simulink library "qrd_matrix_library"  (Simulink 8.7)
settings: Solver=ode45  StartTime=0.0  StopTime=10.0  RelTol=1e-3
values from neighbouring files (symbols this model uses):
  vectorization = 2    [qrd_test.m]
undefined symbols (not defined in the file or in its folder): AdvDSPBChannelOutDisplay, AdvDSPBDMemDisplay, Back_Substitution_instances, column_count, column_count_1, column_count_2, dpoly, dspba_ChannelInVis, dspba_ChannelOutVis, dspba_internal_get_channel_ports, evalAionMaskParam, latency, primtype, QRD_vectorization, recipsqrt, row, row_count, row_count_1, row_count_2, UseDontCare, value, x
libraries: DSPBAPrim x683, DSPBAControl x37, qrd_matrix_library x33, DSPBAVectorUtil x6, DSPBAVectorPrim x3
(part 8 of 8)

== system qrd_matrix_library/matrix_inversion/Z_Address_Gen ==
  Valid_In : Inport
  Channel_In : Inport  Port=2
  Minor_Index : Inport  Port=3
  Major_Index : Inport  Port=4
  size : Inport  Port=5
  SOP_In : Inport  Port=6
  EOP_In : Inport  Port=7
  Add : DSPBAPrim/Add  primtype=add  nInputs=evalAionMaskParam(gcb,'value',1)  nOutputs=1  omode=Specify via dialog  otype=uint(nextpow2(size*size/vectorization))  scale=1  rndmethod=Unbiased  factor=1  satmethod=Symmetric  shift_vec=[0 1 2 -1]  value=2  inPortNames=[' '; ' ';]  outPortNames=[' ']  dspbaimage=dspba_prim.jpg  text=fprintf('+');  style=Optimised  visibilities=1032+2^17+2^18+2^19  genFPC=off  floatRounding=correct  advOptions=[]  version=20130821
  ChannelIn : DSPBAPrim/ChannelIn  primtype=channelin  nInputs=dspba_internal_get_channel_ports(gcb)  nOutputs=dspba_internal_get_channel_ports(gcb)  omode=Inherit via internal rule  otype=sfix(16)  scale=2^-15  rndmethod=Unbiased  factor=1  satmethod=Symmetric  shift_vec=[0 1 2 -1]  value=5  inPortNames=['v'; 'c'; '0'; '1'; '2'; '3'; '4'; '5'; '6'; '7'; '8'; '9'; 'A'; 'B'; 'D'; 'E'; 'F'; 'G'; 'H'; 'I'; 'J'; 'K'; 'L'; 'M'; 'N'; 'O'; 'P'; 'Q'; 'R'; 'S'; 'T'; 'U'; 'W'; 'X'; 'Y'; 'Z']  outPortNames=['v'; 'c'; '0'; '1'; '2'; '3'; '4'; '5'; '6'; '7'; '8'; '9'; 'A'; 'B'; 'D'; 'E'; 'F'; 'G'; 'H'; 'I'; 'J'; 'K'; 'L'; 'M'; 'N'; 'O'; 'P'; 'Q'; 'R'; 'S'; 'T'; 'U'; 'W'; 'X'; 'Y'; 'Z']  dspbaimage=dspba_prim.jpg  text=fprintf('In');  style=Optimised  dataSignals=5  foldingEnabled=off  channels=1  sampleRate=200  packetBeginPresent=off  packetBeginEnabled=off  visibilities=dspba_ChannelInVis(gcb)  latencyCorrection=0  version=20141013
  ChannelOut : DSPBAPrim/ChannelOut  primtype=channelout  nInputs=dspba_internal_get_channel_ports(gcb)  nOutputs=dspba_internal_get_channel_ports(gcb)  omode=Inherit via internal rule  otype=sfix(16)  scale=2^-15  rndmethod=Unbiased  factor=1  satmethod=Symmetric  shift_vec=[0 1 2 -1]  value=3  inPortNames=['v'; 'c'; '0'; '1'; '2'; '3'; '4'; '5'; '6'; '7'; '8'; '9'; 'A'; 'B'; 'D'; 'E'; 'F'; 'G'; 'H'; 'I'; 'J'; 'K'; 'L'; 'M'; 'N'; 'O'; 'P'; 'Q'; 'R'; 'S'; 'T'; 'U'; 'W'; 'X'; 'Y'; 'Z']  outPortNames=['v'; 'c'; '0'; '1'; '2'; '3'; '4'; '5'; '6'; '7'; '8'; '9'; 'A'; 'B'; 'D'; 'E'; 'F'; 'G'; 'H'; 'I'; 'J'; 'K'; 'L'; 'M'; 'N'; 'O'; 'P'; 'Q'; 'R'; 'S'; 'T'; 'U'; 'W'; 'X'; 'Y'; 'Z']  dspbaimage=dspba_prim.jpg  text=fprintf('Out%s', AdvDSPBChannelOutDisplay(latency));  style=Optimised  dataSignals=3  foldingEnabled=off  channels=1  sampleRate=200  packetBeginPresent=off  packetBeginEnabled=off  visibilities=dspba_ChannelOutVis(gcb)  latency=0  latencyCorrection=0  version=20141013
  Mult : DSPBAPrim/Mult  primtype=mult  nInputs=2  nOutputs=1  omode=Inherit via internal rule  otype=sfix(16)  scale=2^-15  rndmethod=Unbiased  factor=1  satmethod=Symmetric  shift_vec=[0 1 2 -1]  value=0  inPortNames=[' '; ' ';]  outPortNames=[' ']  dspbaimage=dspba_prim.jpg  text=fprintf('X');  style=Optimised  visibilities=8+2^18+2^19  floatPrecision=float32_m23  floatRounding=correct  advOptions=[]  version=20130115
  SynthesisInfo : DSPBAPrim/SynthesisInfo  primtype=synthinfo  nInputs=0  nOutputs=0  omode=Inherit via internal rule  otype=sfix(16)  scale=2^-15  rndmethod=Truncate  factor=1  satmethod=Symmetric  shift_vec=[0 1 2 -1]  value=99  inPortNames=[' '; ' ';]  outPortNames=[' ']  dspbaimage=dspba_prim_ctrl.jpg  text=fprintf('Style=%s', style);  style=Scheduled  visibilities=32768  constraintInUse=off  constraintRelation=>  constraintLimit=2  bitAccurate=off  version=20150220
  Valid_Out : Outport
  Channel_Out : Outport  Port=2
  Read_Address : Outport  Port=3
  SOP_Out : Outport  Port=4
  EOP_Out : Outport  Port=5
  wires:
  ChannelIn/2 -> ChannelOut/2
  ChannelOut/5 -> EOP_Out/1
  ChannelOut/4 -> SOP_Out/1
  EOP_In/1 -> ChannelIn/7
  SOP_In/1 -> ChannelIn/6
  ChannelIn/7 -> ChannelOut/5
  ChannelIn/6 -> ChannelOut/4
  Add/1 -> ChannelOut/3
  ChannelIn/5 -> Mult/2
  size/1 -> ChannelIn/5
  Major_Index/1 -> ChannelIn/4
  ChannelOut/2 -> Channel_Out/1
  ChannelOut/3 -> Read_Address/1
  ChannelOut/1 -> Valid_Out/1
  ChannelIn/3 -> Mult/1
  Mult/1 -> Add/2
  ChannelIn/1 -> ChannelOut/1
  Channel_In/1 -> ChannelIn/2
  Minor_Index/1 -> ChannelIn/3
  Valid_In/1 -> ChannelIn/1
  ChannelIn/4 -> Add/1

== system qrd_matrix_library/matrix_inversion/vectorizer ==
  Valid_In : Inport
  Channel_In : Inport  Port=2
  Data_In : Inport  Port=3
  SOP_In : Inport  Port=4
  EOP_In : Inport  Port=5
  ChannelIn : DSPBAPrim/ChannelIn  Commented=on  primtype=channelin  nInputs=dspba_internal_get_channel_ports(gcb)  nOutputs=dspba_internal_get_channel_ports(gcb)  omode=Inherit via internal rule  otype=sfix(16)  scale=2^-15  rndmethod=Unbiased  factor=1  satmethod=Symmetric  shift_vec=[0 1 2 -1]  value=3  inPortNames=['v'; 'c'; '0'; '1'; '2'; '3'; '4'; '5'; '6'; '7'; '8'; '9'; 'A'; 'B'; 'D'; 'E'; 'F'; 'G'; 'H'; 'I'; 'J'; 'K'; 'L'; 'M'; 'N'; 'O'; 'P'; 'Q'; 'R'; 'S'; 'T'; 'U'; 'W'; 'X'; 'Y'; 'Z']  outPortNames=['v'; 'c'; '0'; '1'; '2'; '3'; '4'; '5'; '6'; '7'; '8'; '9'; 'A'; 'B'; 'D'; 'E'; 'F'; 'G'; 'H'; 'I'; 'J'; 'K'; 'L'; 'M'; 'N'; 'O'; 'P'; 'Q'; 'R'; 'S'; 'T'; 'U'; 'W'; 'X'; 'Y'; 'Z']  dspbaimage=dspba_prim.jpg  text=fprintf('In');  style=Optimised  dataSignals=3  foldingEnabled=off  channels=1  sampleRate=200  packetBeginPresent=off  packetBeginEnabled=off  visibilities=dspba_ChannelInVis(gcb)  latencyCorrection=0  version=20141013
  ChannelOut : DSPBAPrim/ChannelOut  Commented=on  primtype=channelout  nInputs=dspba_internal_get_channel_ports(gcb)  nOutputs=dspba_internal_get_channel_ports(gcb)  omode=Inherit via internal rule  otype=sfix(16)  scale=2^-15  rndmethod=Unbiased  factor=1  satmethod=Symmetric  shift_vec=[0 1 2 -1]  value=3  inPortNames=['v'; 'c'; '0'; '1'; '2'; '3'; '4'; '5'; '6'; '7'; '8'; '9'; 'A'; 'B'; 'D'; 'E'; 'F'; 'G'; 'H'; 'I'; 'J'; 'K'; 'L'; 'M'; 'N'; 'O'; 'P'; 'Q'; 'R'; 'S'; 'T'; 'U'; 'W'; 'X'; 'Y'; 'Z']  outPortNames=['v'; 'c'; '0'; '1'; '2'; '3'; '4'; '5'; '6'; '7'; '8'; '9'; 'A'; 'B'; 'D'; 'E'; 'F'; 'G'; 'H'; 'I'; 'J'; 'K'; 'L'; 'M'; 'N'; 'O'; 'P'; 'Q'; 'R'; 'S'; 'T'; 'U'; 'W'; 'X'; 'Y'; 'Z']  dspbaimage=dspba_prim.jpg  text=fprintf('Out%s', AdvDSPBChannelOutDisplay(latency));  style=Optimised  dataSignals=3  foldingEnabled=off  channels=1  sampleRate=200  packetBeginPresent=off  packetBeginEnabled=off  visibilities=dspba_ChannelOutVis(gcb)  latency=0  latencyCorrection=0  version=20141013
  CmpEQ : DSPBAPrim/CmpEQ  primtype=cmpeq  nInputs=2  nOutputs=1  omode=boolean  otype=sfix(16)  scale=2^-15  rndmethod=Unbiased  factor=1  satmethod=Symmetric  shift_vec=[0 1 2 -1]  value=0  inPortNames=[' '; ' ';]  outPortNames=[' ']  dspbaimage=dspba_prim.jpg  text=fprintf('==');  style=Optimised  visibilities=0  advOptions=[]  version=20130117
  Const1 : DSPBAPrim/Const  primtype=const  nInputs=0  nOutputs=1  omode=Inherit via internal rule  otype=uint(8)  scale=1  rndmethod=Unbiased  factor=1  satmethod=Symmetric  shift_vec=[0 1 2 -1]  value=1  inPortNames=['+'; '+';]  outPortNames=[' ']  dspbaimage=dspba_prim.jpg  text=fprintf('%s', num2str(value));  style=Optimised  visibilities=8 + 1024  floatPrecision=float32_m23  version=20120820
  Const11 : DSPBAPrim/Const  primtype=const  nInputs=0  nOutputs=1  omode=Inherit via internal rule  otype=uint(8)  scale=1  rndmethod=Unbiased  factor=1  satmethod=Symmetric  shift_vec=[0 1 2 -1]  value=Back_Substitution_instances/QRD_vectorization  inPortNames=['+'; '+';]  outPortNames=[' ']  dspbaimage=dspba_prim.jpg  text=fprintf('%s', num2str(value));  style=Optimised  visibilities=8 + 1024  floatPrecision=float32_m23  version=20120820
  Const2 : DSPBAPrim/Const  primtype=const  nInputs=0  nOutputs=1  omode=Inherit via internal rule  otype=uint(8)  scale=1  rndmethod=Unbiased  factor=1  satmethod=Symmetric  shift_vec=[0 1 2 -1]  value=(Back_Substitution_instances/QRD_vectorization)-1  inPortNames=['+'; '+';]  outPortNames=[' ']  dspbaimage=dspba_prim.jpg  text=fprintf('%s', num2str(value));  style=Optimised  visibilities=8 + 1024  floatPrecision=float32_m23  version=20120820
  Const8 : DSPBAPrim/Const  primtype=const  nInputs=0  nOutputs=1  omode=Inherit via internal rule  otype=uint(8)  scale=1  rndmethod=Unbiased  factor=1  satmethod=Symmetric  shift_vec=[0 1 2 -1]  value=0  inPortNames=['+'; '+';]  outPortNames=[' ']  dspbaimage=dspba_prim.jpg  text=fprintf('%s', num2str(value));  style=Optimised  visibilities=8 + 1024  floatPrecision=float32_m23  version=20120820
  LoadableCounter : DSPBAPrim/LoadableCounter  primtype=loadablecounter  nInputs=5  nOutputs=1  omode=Inherit via internal rule  otype=ufix(16)  scale=2^-0  rndmethod=Unbiased  factor=1  satmethod=Symmetric  shift_vec=[0 1 2 -1]  value=[0 (Back_Substitution_instances/QRD_vectorization) 0]  inPortNames=['en';'ld';'i ';'s ';'m ']  outPortNames=[' ']  dspbaimage=dspba_prim.jpg  text=fprintf('loadable\ncounter\n[%d %d %d]', value(1), value(2), value(3));  style=Optimised  visibilities=8 + 1024  version=20090407
  SynthesisInfo : DSPBAPrim/SynthesisInfo  Commented=on  primtype=synthinfo  nInputs=0  nOutputs=0  omode=Inherit via internal rule  otype=sfix(16)  scale=2^-15  rndmethod=Truncate  factor=1  satmethod=Symmetric  shift_vec=[0 1 2 -1]  value=99  inPortNames=[' '; ' ';]  outPortNames=[' ']  dspbaimage=dspba_prim_ctrl.jpg  text=fprintf('Style=%s', style);  style=Scheduled  visibilities=2^17+2^18+2^19+2^20  constraintInUse=off  constraintRelation=>  constraintLimit=2  bitAccurate=off  version=20150220
  TappedDelay : qrd_matrix_library/TappedDelay  numTaps=Back_Substitution_instances/QRD_vectorization
  cmp_delay{,1..4} (5 alike) : DSPBAPrim/SampleDelay  primtype=sampdelay  nInputs=1  nOutputs=1  omode=Inherit via internal rule  otype=sfix(16)  scale=2^-15  rndmethod=Unbiased  factor=1  satmethod=Symmetric  shift_vec=[0 1 2 -1]  value=1  inPortNames=[' '; ' ';]  outPortNames=[' ']  dspbaimage=dspba_prim.jpg  text=dpoly(1, eye(1,value+1), 'z')  style=Optimised  visibilities=8 + 1024 + 2^17 + 2^18  flexible=off  slackgroup=0  augmented=0  version=20090407  advOptions=[]
  cntdelay{,1..4} (5 alike) : DSPBAPrim/SampleDelay  primtype=sampdelay  nInputs=1  nOutputs=1  omode=Inherit via internal rule  otype=sfix(16)  scale=2^-15  rndmethod=Unbiased  factor=1  satmethod=Symmetric  shift_vec=[0 1 2 -1]  value=(Back_Substitution_instances/QRD_vectorization)-1  inPortNames=[' '; ' ';]  outPortNames=[' ']  dspbaimage=dspba_prim.jpg  text=dpoly(1, eye(1,value+1), 'z')  style=Optimised  visibilities=8 + 1024 + 2^17 + 2^18  flexible=off  slackgroup=0  augmented=0  version=20090407  advOptions=[]
  sop_delay : DSPBAPrim/SampleDelay  primtype=sampdelay  nInputs=1  nOutputs=1  omode=Inherit via internal rule  otype=sfix(16)  scale=2^-15  rndmethod=Unbiased  factor=1  satmethod=Symmetric  shift_vec=[0 1 2 -1]  value=(Back_Substitution_instances/QRD_vectorization)-1  inPortNames=[' '; ' ';]  outPortNames=[' ']  dspbaimage=dspba_prim.jpg  text=dpoly(1, eye(1,value+1), 'z')  style=Optimised  visibilities=8 + 1024 + 2^17 + 2^18  flexible=off  slackgroup=0  augmented=0  version=20090407  advOptions=[]
  Valid_Out : Outport
  Channel_Out : Outport  Port=2
  Data_Out : Outport  Port=3
  SOP_Out : Outport  Port=4
  EOP_Out : Outport  Port=5
  wires:
  CmpEQ/1 -> cmp_delay/1
  TappedDelay/1 -> cmp_delay2/1
  cntdelay4/1 -> cmp_delay4/1
  cntdelay1/1 -> cmp_delay1/1
  cntdelay3/1 -> sop_delay/1
  LoadableCounter/1 -> CmpEQ/1
  Valid_In/1 -> cntdelay/1
  Channel_In/1 -> cntdelay1/1
  Data_In/1 -> cntdelay2/1
  SOP_In/1 -> cntdelay3/1, LoadableCounter/2
  EOP_In/1 -> cntdelay4/1
  Const1/1 -> LoadableCounter/4
  Const8/1 -> LoadableCounter/3
  Const11/1 -> LoadableCounter/5
  Const2/1 -> CmpEQ/2
  cmp_delay/1 -> Valid_Out/1
  cmp_delay1/1 -> Channel_Out/1
  cmp_delay2/1 -> Data_Out/1
  cmp_delay3/1 -> SOP_Out/1
  cmp_delay4/1 -> EOP_Out/1
  cntdelay2/1 -> TappedDelay/1
  cntdelay/1 -> LoadableCounter/1
  sop_delay/1 -> cmp_delay3/1

== system qrd_matrix_library/matrix_multiplication/Control Logic ==
  Input Valid 1 : Inport
  Input SOP 1 : Inport  Port=2
  Input Valid 2 : Inport  Port=3
  Input SOP 2 : Inport  Port=4
  row1 : Inport  Port=5
  column1 : Inport  Port=6
  column2 : Inport  Port=7
  Output Idle : Inport  Port=8
  Row Major Control Logic : qrd_matrix_library/Row Major Control Logic
  Start 1 : Outport
  Start 2 : Outport  Port=2
  Input Write Address 1 : Outport  Port=3
  Input Write Address 2 : Outport  Port=4
  Read Address Valid : Outport  Port=5
  Input 1 Read Address : Outport  Port=6
  Input 2 Read Address : Outport  Port=7
  Acc_Init : Outport  Port=8
  Acc_Valid : Outport  Port=9
  Result Address : Outport  Port=10
  Done : Outport  Port=11
  wires:
  Input Valid 1/1 -> Row Major Control Logic/1
  Input SOP 1/1 -> Row Major Control Logic/2
  Input Valid 2/1 -> Row Major Control Logic/3
  Input SOP 2/1 -> Row Major Control Logic/4
  row1/1 -> Row Major Control Logic/5
  column1/1 -> Row Major Control Logic/6
  column2/1 -> Row Major Control Logic/7
  Output Idle/1 -> Row Major Control Logic/8
  Row Major Control Logic/1 -> Start 1/1
  Row Major Control Logic/2 -> Start 2/1
  Row Major Control Logic/3 -> Input Write Address 1/1
  Row Major Control Logic/4 -> Input Write Address 2/1
  Row Major Control Logic/5 -> Read Address Valid/1
  Row Major Control Logic/6 -> Input 1 Read Address/1
  Row Major Control Logic/7 -> Input 2 Read Address/1
  Row Major Control Logic/8 -> Acc_Init/1
  Row Major Control Logic/9 -> Acc_Valid/1
  Row Major Control Logic/10 -> Result Address/1
  Row Major Control Logic/11 -> Done/1

== system qrd_matrix_library/matrix_multiplication/Input Memory Controller ==
  External Write 1 : Inport
  External Write Address 1 : Inport  Port=2
  External Write Data 1 : Inport  Port=3
  Read Address 1 : Inport  Port=4
  External Write 2 : Inport  Port=5
  External Write Address 2 : Inport  Port=6
  External Write Data 2 : Inport  Port=7
  Read Address 2 : Inport  Port=8
  Input RAM 1 : DSPBAPrim/DualMem  primtype=dualmem  nInputs=4  nOutputs=2  omode=Inherit via internal rule  otype=sfix(16)  scale=2^-15  rndmethod=Unbiased  factor=1  satmethod=Symmetric  shift_vec=[0 1 2 -1]  value=complex(zeros((row_count_1*column_count_1)/vectorization,vectorization),zeros((row_count_1*column_count_1)/vectorization,vectorization))  inPortNames=['d1'; 'a1'; 'w1'; 'a2']  outPortNames=['q1'; 'q2']  dspbaimage=dspba_prim.jpg  text=fprintf('dmem%s',AdvDSPBDMemDisplay(UseDontCare));  style=Optimised  visibilities=8 + 1024 + 2^17 + 2^18  UseDontCare=off  TwinWritePorts=off  version=20141001
  Input RAM 2 : DSPBAPrim/DualMem  primtype=dualmem  nInputs=4  nOutputs=2  omode=Inherit via internal rule  otype=sfix(16)  scale=2^-15  rndmethod=Unbiased  factor=1  satmethod=Symmetric  shift_vec=[0 1 2 -1]  value=complex(zeros((row_count_2*column_count_2)/vectorization,vectorization),zeros((row_count_2*column_count_2)/vectorization,vectorization))  inPortNames=['d1'; 'a1'; 'w1'; 'a2']  outPortNames=['q1'; 'q2']  dspbaimage=dspba_prim.jpg  text=fprintf('dmem%s',AdvDSPBDMemDisplay(UseDontCare));  style=Optimised  visibilities=8 + 1024 + 2^17 + 2^18  UseDontCare=off  TwinWritePorts=off  version=20141001
  Data 1 : Outport
  Data 2 : Outport  Port=2
  wires:
  Read Address 1/1 -> Input RAM 1/4
  External Write Address 1/1 -> Input RAM 1/2
  External Write Data 1/1 -> Input RAM 1/1
  External Write 1/1 -> Input RAM 1/3
  Read Address 2/1 -> Input RAM 2/4
  Input RAM 1/2 -> Data 1/1
  Input RAM 2/2 -> Data 2/1
  External Write 2/1 -> Input RAM 2/3
  External Write Address 2/1 -> Input RAM 2/2
  External Write Data 2/1 -> Input RAM 2/1

== system qrd_matrix_library/matrix_multiplication/MAC ==
  note: Floating Point MAC
  Valid In : Inport
  Channel In : Inport  Port=2
  Input 1 Data : Inport  Port=3
  Input 2 Data : Inport  Port=4
  Acc_Init : Inport  Port=5
  Acc_Valid : Inport  Port=6
  Result Address In : Inport  Port=7
  Done In : Inport  Port=8
  And : DSPBAPrim/And  primtype=and  nInputs=2  nOutputs=1  omode=Inherit via internal rule  otype=sfix(16)  scale=2^-15  rndmethod=Unbiased  factor=1  satmethod=Symmetric  shift_vec=[0 1 2 -1]  value=0  inPortNames=[' '; ' '; ' '; ' '; ' '; ' '; ' '; ' '; ' '; ' '; ' '; ' '; ' '; ' '; ' '; ' '; ]  outPortNames=[' ']  dspbaimage=dspba_prim.jpg  text=fprintf('&');  style=Optimised  visibilities=8+2  version=20090407
  ChannelIn : DSPBAPrim/ChannelIn  primtype=channelin  nInputs=dspba_internal_get_channel_ports(gcb)  nOutputs=dspba_internal_get_channel_ports(gcb)  omode=Inherit via internal rule  otype=sfix(16)  scale=2^-15  rndmethod=Unbiased  factor=1  satmethod=Symmetric  shift_vec=[0 1 2 -1]  value=6  inPortNames=['v'; 'c'; '0'; '1'; '2'; '3'; '4'; '5'; '6'; '7'; '8'; '9'; 'A'; 'B'; 'D'; 'E'; 'F'; 'G'; 'H'; 'I'; 'J'; 'K'; 'L'; 'M'; 'N'; 'O'; 'P'; 'Q'; 'R'; 'S'; 'T'; 'U'; 'W'; 'X'; 'Y'; 'Z']  outPortNames=['v'; 'c'; '0'; '1'; '2'; '3'; '4'; '5'; '6'; '7'; '8'; '9'; 'A'; 'B'; 'D'; 'E'; 'F'; 'G'; 'H'; 'I'; 'J'; 'K'; 'L'; 'M'; 'N'; 'O'; 'P'; 'Q'; 'R'; 'S'; 'T'; 'U'; 'W'; 'X'; 'Y'; 'Z']  dspbaimage=dspba_prim.jpg  text=fprintf('In');  style=Optimised  dataSignals=6  foldingEnabled=off  channels=1  sampleRate=200  packetBeginPresent=off  packetBeginEnabled=off  visibilities=dspba_ChannelInVis(gcb)  latencyCorrection=0  version=20141013
  ChannelOut : DSPBAPrim/ChannelOut  primtype=channelout  nInputs=dspba_internal_get_channel_ports(gcb)  nOutputs=dspba_internal_get_channel_ports(gcb)  omode=Inherit via internal rule  otype=sfix(16)  scale=2^-15  rndmethod=Unbiased  factor=1  satmethod=Symmetric  shift_vec=[0 1 2 -1]  value=3  inPortNames=['v'; 'c'; '0'; '1'; '2'; '3'; '4'; '5'; '6'; '7'; '8'; '9'; 'A'; 'B'; 'D'; 'E'; 'F'; 'G'; 'H'; 'I'; 'J'; 'K'; 'L'; 'M'; 'N'; 'O'; 'P'; 'Q'; 'R'; 'S'; 'T'; 'U'; 'W'; 'X'; 'Y'; 'Z']  outPortNames=['v'; 'c'; '0'; '1'; '2'; '3'; '4'; '5'; '6'; '7'; '8'; '9'; 'A'; 'B'; 'D'; 'E'; 'F'; 'G'; 'H'; 'I'; 'J'; 'K'; 'L'; 'M'; 'N'; 'O'; 'P'; 'Q'; 'R'; 'S'; 'T'; 'U'; 'W'; 'X'; 'Y'; 'Z']  dspbaimage=dspba_prim.jpg  text=fprintf('Out%s', AdvDSPBChannelOutDisplay(latency));  style=Optimised  dataSignals=3  foldingEnabled=off  channels=1  sampleRate=200  packetBeginPresent=off  packetBeginEnabled=off  visibilities=dspba_ChannelOutVis(gcb)  latency=7  latencyCorrection=0  version=20141013
  Complex to Real-Imag : ComplexToRealImag
  Complex to Real-Imag Transpose : ComplexToRealImag
  Const4 : DSPBAPrim/Const  primtype=const  nInputs=0  nOutputs=1  omode=Inherit via internal rule  otype=uint(8)  scale=1  rndmethod=Unbiased  factor=1  satmethod=Symmetric  shift_vec=[0 1 2 -1]  value=0  inPortNames=['+'; '+';]  outPortNames=[' ']  dspbaimage=dspba_prim.jpg  text=fprintf('%s', num2str(value));  style=Optimised  visibilities=8 + 1024  floatPrecision=float32_m23  version=20120820
  MultAcc ac : DSPBAPrim/MultAcc  primtype=multaccfunc  nInputs=3  nOutputs=1  omode=Inherit via internal rule  otype=sfix(16)  scale=2^-15  rndmethod=Unbiased  factor=1  satmethod=Symmetric  shift_vec=[0 1 2 -1]  value=0  inPortNames="[ 'acc'; 'x  '; 'y  ']"  outPortNames=[]  dspbaimage=dspba_prim_float.jpg  text=disp('multAcc');  style=Optimised  visibilities=8+2^17  functionExpr=fpMultAcc  advOptions=[]  version=20121130
  MultAcc ad : DSPBAPrim/MultAcc  primtype=multaccfunc  nInputs=3  nOutputs=1  omode=Inherit via internal rule  otype=sfix(16)  scale=2^-15  rndmethod=Unbiased  factor=1  satmethod=Symmetric  shift_vec=[0 1 2 -1]  value=0  inPortNames="[ 'acc'; 'x  '; 'y  ']"  outPortNames=[]  dspbaimage=dspba_prim_float.jpg  text=disp('multAcc');  style=Optimised  visibilities=8+2^17  functionExpr=fpMultAcc  advOptions=[]  version=20121130
  MultAcc bc : DSPBAPrim/MultAcc  primtype=multaccfunc  nInputs=3  nOutputs=1  omode=Inherit via internal rule  otype=sfix(16)  scale=2^-15  rndmethod=Unbiased  factor=1  satmethod=Symmetric  shift_vec=[0 1 2 -1]  value=0  inPortNames="[ 'acc'; 'x  '; 'y  ']"  outPortNames=[]  dspbaimage=dspba_prim_float.jpg  text=disp('multAcc');  style=Optimised  visibilities=8+2^17  functionExpr=fpMultAcc  advOptions=[]  version=20121130
  MultAcc bd : DSPBAPrim/MultAcc  primtype=multaccfunc  nInputs=3  nOutputs=1  omode=Inherit via internal rule  otype=sfix(16)  scale=2^-15  rndmethod=Unbiased  factor=1  satmethod=Symmetric  shift_vec=[0 1 2 -1]  value=0  inPortNames="[ 'acc'; 'x  '; 'y  ']"  outPortNames=[]  dspbaimage=dspba_prim_float.jpg  text=disp('multAcc');  style=Optimised  visibilities=8+2^17  functionExpr=fpMultAcc  advOptions=[]  version=20121130
  Not : DSPBAPrim/Not  primtype=not  nInputs=1  nOutputs=1  omode=Inherit via internal rule  otype=sfix(16)  scale=2^-15  rndmethod=Unbiased  factor=1  satmethod=Symmetric  shift_vec=[0 1 2 -1]  value=0  inPortNames=[' '; ' ';]  outPortNames=[' ']  dspbaimage=dspba_prim.jpg  text=fprintf('~');  style=Optimised  visibilities=8  version=20090407
  Real-Imag to Complex : RealImagToComplex
  SumOfElements : DSPBAVectorPrim/SumOfElements  primtype=sumofelements  nInputs=1  nOutputs=1  omode=Inherit via internal rule with word growth  otype=sfix(16)  scale=2^-15  rndmethod=Unbiased  factor=1  satmethod=Symmetric  shift_vec=[0 1 2 -1]  value=1  inPortNames=[' '; ' ';]  outPortNames=[' ']  dspbaimage=dspba_prim.jpg  text=fprintf('+');  style=Optimised  visibilities=8+2^17+2^18+2^19  genFPC=off  floatRounding=correct  advOptions=[]  version=20130821
  SynthesisInfo : DSPBAPrim/SynthesisInfo  primtype=synthinfo  nInputs=0  nOutputs=0  omode=Inherit via internal rule  otype=sfix(16)  scale=2^-15  rndmethod=Truncate  factor=1  satmethod=Symmetric  shift_vec=[0 1 2 -1]  value=99  inPortNames=[' '; ' ';]  outPortNames=[' ']  dspbaimage=dspba_prim_ctrl.jpg  text=fprintf('Style=%s', style);  style=Scheduled  visibilities=2^17+2^18+2^19+2^20  constraintInUse=off  constraintRelation=>  constraintLimit=2  bitAccurate=off  version=20150220
  ac-bd : DSPBAPrim/Sub  primtype=sub  nInputs=2  nOutputs=1  omode=Inherit via internal rule with word growth  otype=sfix(16)  scale=2^-15  rndmethod=Unbiased  factor=1  satmethod=Symmetric  shift_vec=[0 1 2 -1]  value=0  inPortNames=['+'; '-';]  outPortNames=[' ']  dspbaimage=dspba_prim.jpg  text=fprintf('-');  style=Optimised  visibilities=8+2^17+2^18  floatRounding=correct  advOptions=[]  version=20130115
  bc+ad : DSPBAPrim/Add  primtype=add  nInputs=evalAionMaskParam(gcb,'value',1)  nOutputs=1  omode=Inherit via internal rule with word growth  otype=sfix(16)  scale=2^-15  rndmethod=Unbiased  factor=1  satmethod=Symmetric  shift_vec=[0 1 2 -1]  value=2  inPortNames=[' '; ' ';]  outPortNames=[' ']  dspbaimage=dspba_prim.jpg  text=fprintf('+');  style=Optimised  visibilities=1032+2^17+2^18+2^19  genFPC=off  floatRounding=correct  advOptions=[]  version=20130821
  Valid Out : Outport
  Result Data : Outport  Port=2
  Result Address Out : Outport  Port=3
  Done Out : Outport  Port=4
  wires:
  Input 1 Data/1 -> ChannelIn/3
  Acc_Valid/1 -> ChannelIn/6
  Input 2 Data/1 -> ChannelIn/4
  Valid In/1 -> ChannelIn/1
  Result Address In/1 -> ChannelIn/7
  Acc_Init/1 -> ChannelIn/5
  Channel In/1 -> ChannelIn/2
  ChannelIn/5 -> Not/1
  Real-Imag to Complex/1 -> SumOfElements/1
  ChannelIn/1 -> And/1
  And/1 -> ChannelOut/1
  ChannelIn/6 -> And/2
  ChannelIn/7 -> [Result_Address]
  ChannelOut/3 -> Result Data/1
  ChannelOut/4 -> Result Address Out/1
  ChannelOut/5 -> Done Out/1
  Done In/1 -> ChannelIn/8
  ChannelIn/8 -> [Done]
  MultAcc ad/1 -> bc+ad/2  "ad"
  MultAcc bc/1 -> bc+ad/1  "bc"
  Complex to Real-Imag Transpose/2 -> MultAcc ad/3, MultAcc bd/3  "d"
  Complex to Real-Imag Transpose/1 -> MultAcc ac/3, MultAcc bc/3  "c"
  ChannelIn/3 -> Complex to Real-Imag/1
  ChannelIn/4 -> Complex to Real-Imag Transpose/1
  Complex to Real-Imag/2 -> MultAcc bc/2, MultAcc bd/2  "b"
  MultAcc bd/1 -> ac-bd/2  "bd"
  Complex to Real-Imag/1 -> MultAcc ad/2, MultAcc ac/2  "a"
  Not/1 -> MultAcc ad/1, MultAcc bc/1, MultAcc bd/1, MultAcc ac/1
  MultAcc ac/1 -> ac-bd/1  "ac"
  bc+ad/1 -> Real-Imag to Complex/2  "bc+ad"
  ac-bd/1 -> Real-Imag to Complex/1  "ac-bd"
  ChannelOut/1 -> Valid Out/1
  [Result_Address] -> ChannelOut/4
  [Done] -> ChannelOut/5
  Const4/1 -> ChannelOut/2
  SumOfElements/1 -> ChannelOut/3

== system qrd_matrix_library/matrix_multiplication/Output Memory Controller ==
  Write Enable : Inport
  Write Address : Inport  Port=2
  Write Data : Inport  Port=3
  Read Address : Inport  Port=4
  Result RAM : DSPBAPrim/DualMem  primtype=dualmem  nInputs=4  nOutputs=2  omode=Inherit via internal rule  otype=sfix(16)  scale=2^-15  rndmethod=Unbiased  factor=1  satmethod=Symmetric  shift_vec=[0 1 2 -1]  value=complex(zeros(row_count_1*column_count_2,1),zeros(row_count_1*column_count_2,1))  inPortNames=['d1'; 'a1'; 'w1'; 'a2']  outPortNames=['q1'; 'q2']  dspbaimage=dspba_prim.jpg  text=fprintf('dmem%s',AdvDSPBDMemDisplay(UseDontCare));  style=Optimised  visibilities=8 + 1024 + 2^17 + 2^18  UseDontCare=on  TwinWritePorts=off  version=20141001
  Read Data : Outport
  wires:
  Write Address/1 -> Result RAM/2
  Write Data/1 -> Result RAM/1
  Read Address/1 -> Result RAM/4
  Result RAM/2 -> Read Data/1
  Write Enable/1 -> Result RAM/3

== system qrd_matrix_library/matrix_multiplication/Rising Edge Detect ==
  d : Inport
  And : DSPBAPrim/And  primtype=and  nInputs=2  nOutputs=1  omode=Inherit via internal rule  otype=sfix(16)  scale=2^-15  rndmethod=Unbiased  factor=1  satmethod=Symmetric  shift_vec=[0 1 2 -1]  value=0  inPortNames=[' '; ' '; ' '; ' '; ' '; ' '; ' '; ' '; ' '; ' '; ' '; ' '; ' '; ' '; ' '; ' '; ]  outPortNames=[' ']  dspbaimage=dspba_prim.jpg  text=fprintf('&');  style=Optimised  visibilities=8+2  version=20090407
  SampleDelay : DSPBAPrim/SampleDelay  primtype=sampdelay  nInputs=1  nOutputs=1  omode=Inherit via internal rule  otype=sfix(16)  scale=2^-15  rndmethod=Unbiased  factor=1  satmethod=Symmetric  shift_vec=[0 1 2 -1]  value=1  inPortNames=[' '; ' ';]  outPortNames=[' ']  dspbaimage=dspba_prim.jpg  text=dpoly(1, eye(1,value+1), 'z')  style=Optimised  visibilities=8 + 1024 + 2^17 + 2^18  flexible=off  slackgroup=0  augmented=0  version=20090407  advOptions=[]
  Xor : DSPBAPrim/Xor  primtype=xor  nInputs=2  nOutputs=1  omode=Inherit via internal rule  otype=sfix(16)  scale=2^-15  rndmethod=Unbiased  factor=1  satmethod=Symmetric  shift_vec=[0 1 2 -1]  value=0  inPortNames=[' '; ' '; ' '; ' '; ' '; ' '; ' '; ' '; ' '; ' '; ' '; ' '; ' '; ' '; ' '; ' '; ]  outPortNames=[' ']  dspbaimage=dspba_prim.jpg  text=fprintf('^');  style=Optimised  visibilities=8+2  version=20090407
  q : Outport
  wires:
  SampleDelay/1 -> Xor/2
  Xor/1 -> And/1
  d/1 -> And/2, Xor/1, SampleDelay/1
  And/1 -> q/1

== system qrd_matrix_library/QR_decomposition/Control Logic/A_j_Address_Gen ==
  Valid_In : Inport
  Channel_In : Inport  Port=2
  Row_Index : Inport  Port=3
  Column : Inport  Port=4
  Row : Inport  Port=5
  Acc_Init_In : Inport  Port=6
  Acc_Valid_In : Inport  Port=7
  Aj_last_col_update_in : Inport  Port=8
  A_k_Read_Valid3_In : Inport  Port=9
  A_k_Read_Address3_In : Inport  Port=10
  Add : DSPBAPrim/Add  primtype=add  nInputs=evalAionMaskParam(gcb,'value',1)  nOutputs=1  omode=Specify via dialog  otype=uint(nextpow2(size*size/vectorization))  scale=1  rndmethod=Unbiased  factor=1  satmethod=Symmetric  shift_vec=[0 1 2 -1]  value=2  inPortNames=[' '; ' ';]  outPortNames=[' ']  dspbaimage=dspba_prim.jpg  text=fprintf('+');  style=Optimised  visibilities=1032+2^17+2^18+2^19  genFPC=off  floatRounding=correct  advOptions=[]  version=20130821
  ChannelIn : DSPBAPrim/ChannelIn  primtype=channelin  nInputs=dspba_internal_get_channel_ports(gcb)  nOutputs=dspba_internal_get_channel_ports(gcb)  omode=Inherit via internal rule  otype=sfix(16)  scale=2^-15  rndmethod=Unbiased  factor=1  satmethod=Symmetric  shift_vec=[0 1 2 -1]  value=8  inPortNames=['v'; 'c'; '0'; '1'; '2'; '3'; '4'; '5'; '6'; '7'; '8'; '9'; 'A'; 'B'; 'D'; 'E'; 'F'; 'G'; 'H'; 'I'; 'J'; 'K'; 'L'; 'M'; 'N'; 'O'; 'P'; 'Q'; 'R'; 'S'; 'T'; 'U'; 'W'; 'X'; 'Y'; 'Z']  outPortNames=['v'; 'c'; '0'; '1'; '2'; '3'; '4'; '5'; '6'; '7'; '8'; '9'; 'A'; 'B'; 'D'; 'E'; 'F'; 'G'; 'H'; 'I'; 'J'; 'K'; 'L'; 'M'; 'N'; 'O'; 'P'; 'Q'; 'R'; 'S'; 'T'; 'U'; 'W'; 'X'; 'Y'; 'Z']  dspbaimage=dspba_prim.jpg  text=fprintf('In');  style=Optimised  dataSignals=8  foldingEnabled=off  channels=1  sampleRate=200  packetBeginPresent=off  packetBeginEnabled=off  visibilities=dspba_ChannelInVis(gcb)  latencyCorrection=0  version=20141013
  ChannelOut : DSPBAPrim/ChannelOut  primtype=channelout  nInputs=dspba_internal_get_channel_ports(gcb)  nOutputs=dspba_internal_get_channel_ports(gcb)  omode=Inherit via internal rule  otype=sfix(16)  scale=2^-15  rndmethod=Unbiased  factor=1  satmethod=Symmetric  shift_vec=[0 1 2 -1]  value=7  inPortNames=['v'; 'c'; '0'; '1'; '2'; '3'; '4'; '5'; '6'; '7'; '8'; '9'; 'A'; 'B'; 'D'; 'E'; 'F'; 'G'; 'H'; 'I'; 'J'; 'K'; 'L'; 'M'; 'N'; 'O'; 'P'; 'Q'; 'R'; 'S'; 'T'; 'U'; 'W'; 'X'; 'Y'; 'Z']  outPortNames=['v'; 'c'; '0'; '1'; '2'; '3'; '4'; '5'; '6'; '7'; '8'; '9'; 'A'; 'B'; 'D'; 'E'; 'F'; 'G'; 'H'; 'I'; 'J'; 'K'; 'L'; 'M'; 'N'; 'O'; 'P'; 'Q'; 'R'; 'S'; 'T'; 'U'; 'W'; 'X'; 'Y'; 'Z']  dspbaimage=dspba_prim.jpg  text=fprintf('Out%s', AdvDSPBChannelOutDisplay(latency));  style=Optimised  dataSignals=7  foldingEnabled=off  channels=1  sampleRate=200  packetBeginPresent=off  packetBeginEnabled=off  visibilities=dspba_ChannelOutVis(gcb)  latency=0  latencyCorrection=0  version=20141013
  Mult : DSPBAPrim/Mult  primtype=mult  nInputs=2  nOutputs=1  omode=Inherit via internal rule  otype=sfix(16)  scale=2^-15  rndmethod=Unbiased  factor=1  satmethod=Symmetric  shift_vec=[0 1 2 -1]  value=0  inPortNames=[' '; ' ';]  outPortNames=[' ']  dspbaimage=dspba_prim.jpg  text=fprintf('X');  style=Optimised  visibilities=8+2^18+2^19  floatPrecision=float32_m23  floatRounding=correct  advOptions=[]  version=20130115
  SynthesisInfo : DSPBAPrim/SynthesisInfo  primtype=synthinfo  nInputs=0  nOutputs=0  omode=Inherit via internal rule  otype=sfix(16)  scale=2^-15  rndmethod=Truncate  factor=1  satmethod=Symmetric  shift_vec=[0 1 2 -1]  value=99  inPortNames=[' '; ' ';]  outPortNames=[' ']  dspbaimage=dspba_prim_ctrl.jpg  text=fprintf('Style=%s', style);  style=Scheduled  visibilities=32768  constraintInUse=off  constraintRelation=>  constraintLimit=2  bitAccurate=off  version=20150220
  Valid_Out : Outport
  Channel_Out : Outport  Port=2
  A_k_j_Read_Address : Outport  Port=3
  A_k_Read_Address : Outport  Port=4
  Acc_Init_Out : Outport  Port=5
  Acc_Valid_Out : Outport  Port=6
  Aj_last_col_update_out : Outport  Port=7
  A_k_Read_Valid3_Out : Outport  Port=8
  A_k_Read_Address3_Out : Outport  Port=9
  wires:
  ChannelIn/2 -> ChannelOut/2
  ChannelOut/6 -> Acc_Valid_Out/1
  ChannelOut/5 -> Acc_Init_Out/1
  Acc_Valid_In/1 -> ChannelIn/7
  Acc_Init_In/1 -> ChannelIn/6
  ChannelIn/7 -> ChannelOut/6
  ChannelIn/6 -> ChannelOut/5
  Add/1 -> ChannelOut/3
  ChannelIn/5 -> Mult/2
  Row/1 -> ChannelIn/5
  Column/1 -> ChannelIn/4
  ChannelIn/4 -> Mult/1
  ChannelOut/2 -> Channel_Out/1
  ChannelOut/3 -> A_k_j_Read_Address/1
  ChannelOut/1 -> Valid_Out/1
  ChannelIn/3 -> ChannelOut/4, Add/1
  Mult/1 -> Add/2
  ChannelIn/1 -> ChannelOut/1
  Channel_In/1 -> ChannelIn/2
  Row_Index/1 -> ChannelIn/3
  Valid_In/1 -> ChannelIn/1
  ChannelOut/4 -> A_k_Read_Address/1
  ChannelOut/7 -> Aj_last_col_update_out/1
  ChannelOut/8 -> A_k_Read_Valid3_Out/1
  A_k_Read_Valid3_In/1 -> ChannelIn/9
  Aj_last_col_update_in/1 -> ChannelIn/8
  ChannelIn/9 -> ChannelOut/8
  ChannelIn/10 -> ChannelOut/9
  A_k_Read_Address3_In/1 -> ChannelIn/10
  ChannelOut/9 -> A_k_Read_Address3_Out/1
  ChannelIn/8 -> ChannelOut/7

== system qrd_matrix_library/QR_decomposition/Control Logic/A_k_Address_Gen ==
  Valid_In : Inport
  Channel_In : Inport  Port=2
  Row_Index : Inport  Port=3
  Column : Inport  Port=4
  Row : Inport  Port=5
  Acc_Init_In : Inport  Port=6
  Acc_Valid_In : Inport  Port=7
  Add : DSPBAPrim/Add  primtype=add  nInputs=evalAionMaskParam(gcb,'value',1)  nOutputs=1  omode=Specify via dialog  otype=uint(nextpow2(size*size/vectorization))  scale=1  rndmethod=Unbiased  factor=1  satmethod=Symmetric  shift_vec=[0 1 2 -1]  value=2  inPortNames=[' '; ' ';]  outPortNames=[' ']  dspbaimage=dspba_prim.jpg  text=fprintf('+');  style=Optimised  visibilities=1032+2^17+2^18+2^19  genFPC=off  floatRounding=correct  advOptions=[]  version=20130821
  ChannelIn : DSPBAPrim/ChannelIn  primtype=channelin  nInputs=dspba_internal_get_channel_ports(gcb)  nOutputs=dspba_internal_get_channel_ports(gcb)  omode=Inherit via internal rule  otype=sfix(16)  scale=2^-15  rndmethod=Unbiased  factor=1  satmethod=Symmetric  shift_vec=[0 1 2 -1]  value=5  inPortNames=['v'; 'c'; '0'; '1'; '2'; '3'; '4'; '5'; '6'; '7'; '8'; '9'; 'A'; 'B'; 'D'; 'E'; 'F'; 'G'; 'H'; 'I'; 'J'; 'K'; 'L'; 'M'; 'N'; 'O'; 'P'; 'Q'; 'R'; 'S'; 'T'; 'U'; 'W'; 'X'; 'Y'; 'Z']  outPortNames=['v'; 'c'; '0'; '1'; '2'; '3'; '4'; '5'; '6'; '7'; '8'; '9'; 'A'; 'B'; 'D'; 'E'; 'F'; 'G'; 'H'; 'I'; 'J'; 'K'; 'L'; 'M'; 'N'; 'O'; 'P'; 'Q'; 'R'; 'S'; 'T'; 'U'; 'W'; 'X'; 'Y'; 'Z']  dspbaimage=dspba_prim.jpg  text=fprintf('In');  style=Optimised  dataSignals=5  foldingEnabled=off  channels=1  sampleRate=200  packetBeginPresent=off  packetBeginEnabled=off  visibilities=dspba_ChannelInVis(gcb)  latencyCorrection=0  version=20141013
  ChannelOut : DSPBAPrim/ChannelOut  primtype=channelout  nInputs=dspba_internal_get_channel_ports(gcb)  nOutputs=dspba_internal_get_channel_ports(gcb)  omode=Inherit via internal rule  otype=sfix(16)  scale=2^-15  rndmethod=Unbiased  factor=1  satmethod=Symmetric  shift_vec=[0 1 2 -1]  value=4  inPortNames=['v'; 'c'; '0'; '1'; '2'; '3'; '4'; '5'; '6'; '7'; '8'; '9'; 'A'; 'B'; 'D'; 'E'; 'F'; 'G'; 'H'; 'I'; 'J'; 'K'; 'L'; 'M'; 'N'; 'O'; 'P'; 'Q'; 'R'; 'S'; 'T'; 'U'; 'W'; 'X'; 'Y'; 'Z']  outPortNames=['v'; 'c'; '0'; '1'; '2'; '3'; '4'; '5'; '6'; '7'; '8'; '9'; 'A'; 'B'; 'D'; 'E'; 'F'; 'G'; 'H'; 'I'; 'J'; 'K'; 'L'; 'M'; 'N'; 'O'; 'P'; 'Q'; 'R'; 'S'; 'T'; 'U'; 'W'; 'X'; 'Y'; 'Z']  dspbaimage=dspba_prim.jpg  text=fprintf('Out%s', AdvDSPBChannelOutDisplay(latency));  style=Optimised  dataSignals=4  foldingEnabled=off  channels=1  sampleRate=200  packetBeginPresent=off  packetBeginEnabled=off  visibilities=dspba_ChannelOutVis(gcb)  latency=0  latencyCorrection=0  version=20141013
  Mult : DSPBAPrim/Mult  primtype=mult  nInputs=2  nOutputs=1  omode=Inherit via internal rule  otype=sfix(16)  scale=2^-15  rndmethod=Unbiased  factor=1  satmethod=Symmetric  shift_vec=[0 1 2 -1]  value=0  inPortNames=[' '; ' ';]  outPortNames=[' ']  dspbaimage=dspba_prim.jpg  text=fprintf('X');  style=Optimised  visibilities=8+2^18+2^19  floatPrecision=float32_m23  floatRounding=correct  advOptions=[]  version=20130115
  SynthesisInfo : DSPBAPrim/SynthesisInfo  primtype=synthinfo  nInputs=0  nOutputs=0  omode=Inherit via internal rule  otype=sfix(16)  scale=2^-15  rndmethod=Truncate  factor=1  satmethod=Symmetric  shift_vec=[0 1 2 -1]  value=99  inPortNames=[' '; ' ';]  outPortNames=[' ']  dspbaimage=dspba_prim_ctrl.jpg  text=fprintf('Style=%s', style);  style=Scheduled  visibilities=32768  constraintInUse=off  constraintRelation=>  constraintLimit=2  bitAccurate=off  version=20150220
  Valid_Out : Outport
  Channel_Out : Outport  Port=2
  Input_Read_Address : Outport  Port=3
  A_k_Write_Address : Outport  Port=4
  Acc_Init_Out : Outport  Port=5
  Acc_Valid_Out : Outport  Port=6
  wires:
  Valid_In/1 -> ChannelIn/1
  Row_Index/1 -> ChannelIn/3
  Channel_In/1 -> ChannelIn/2
  ChannelIn/1 -> ChannelOut/1
  Mult/1 -> Add/2
  ChannelIn/3 -> Add/1, ChannelOut/4
  ChannelOut/1 -> Valid_Out/1
  ChannelOut/3 -> Input_Read_Address/1
  ChannelOut/2 -> Channel_Out/1
  ChannelIn/4 -> Mult/1
  Column/1 -> ChannelIn/4
  Row/1 -> ChannelIn/5
  ChannelIn/5 -> Mult/2
  Add/1 -> ChannelOut/3
  ChannelIn/6 -> ChannelOut/5
  ChannelIn/7 -> ChannelOut/6
  Acc_Init_In/1 -> ChannelIn/6
  Acc_Valid_In/1 -> ChannelIn/7
  ChannelOut/5 -> Acc_Init_Out/1
  ChannelOut/6 -> Acc_Valid_Out/1
  ChannelOut/4 -> A_k_Write_Address/1
  ChannelIn/2 -> ChannelOut/2

== system qrd_matrix_library/QR_decomposition/Control Logic/rn_k_j_Address_Gen ==
  Valid_In : Inport
  Channel_In : Inport  Port=2
  Row_Index : Inport  Port=3
  Column : Inport  Port=4
  Row : Inport  Port=5
  Acc_Init_In : Inport  Port=6
  Acc_Valid_In : Inport  Port=7
  Add : DSPBAPrim/Add  primtype=add  nInputs=evalAionMaskParam(gcb,'value',1)  nOutputs=1  omode=Specify via dialog  otype=uint(nextpow2(size*size/vectorization))  scale=1  rndmethod=Unbiased  factor=1  satmethod=Symmetric  shift_vec=[0 1 2 -1]  value=2  inPortNames=[' '; ' ';]  outPortNames=[' ']  dspbaimage=dspba_prim.jpg  text=fprintf('+');  style=Optimised  visibilities=1032+2^17+2^18+2^19  genFPC=off  floatRounding=correct  advOptions=[]  version=20130821
  ChannelIn : DSPBAPrim/ChannelIn  primtype=channelin  nInputs=dspba_internal_get_channel_ports(gcb)  nOutputs=dspba_internal_get_channel_ports(gcb)  omode=Inherit via internal rule  otype=sfix(16)  scale=2^-15  rndmethod=Unbiased  factor=1  satmethod=Symmetric  shift_vec=[0 1 2 -1]  value=5  inPortNames=['v'; 'c'; '0'; '1'; '2'; '3'; '4'; '5'; '6'; '7'; '8'; '9'; 'A'; 'B'; 'D'; 'E'; 'F'; 'G'; 'H'; 'I'; 'J'; 'K'; 'L'; 'M'; 'N'; 'O'; 'P'; 'Q'; 'R'; 'S'; 'T'; 'U'; 'W'; 'X'; 'Y'; 'Z']  outPortNames=['v'; 'c'; '0'; '1'; '2'; '3'; '4'; '5'; '6'; '7'; '8'; '9'; 'A'; 'B'; 'D'; 'E'; 'F'; 'G'; 'H'; 'I'; 'J'; 'K'; 'L'; 'M'; 'N'; 'O'; 'P'; 'Q'; 'R'; 'S'; 'T'; 'U'; 'W'; 'X'; 'Y'; 'Z']  dspbaimage=dspba_prim.jpg  text=fprintf('In');  style=Optimised  dataSignals=5  foldingEnabled=off  channels=1  sampleRate=200  packetBeginPresent=off  packetBeginEnabled=off  visibilities=dspba_ChannelInVis(gcb)  latencyCorrection=0  version=20141013
  ChannelOut : DSPBAPrim/ChannelOut  primtype=channelout  nInputs=dspba_internal_get_channel_ports(gcb)  nOutputs=dspba_internal_get_channel_ports(gcb)  omode=Inherit via internal rule  otype=sfix(16)  scale=2^-15  rndmethod=Unbiased  factor=1  satmethod=Symmetric  shift_vec=[0 1 2 -1]  value=4  inPortNames=['v'; 'c'; '0'; '1'; '2'; '3'; '4'; '5'; '6'; '7'; '8'; '9'; 'A'; 'B'; 'D'; 'E'; 'F'; 'G'; 'H'; 'I'; 'J'; 'K'; 'L'; 'M'; 'N'; 'O'; 'P'; 'Q'; 'R'; 'S'; 'T'; 'U'; 'W'; 'X'; 'Y'; 'Z']  outPortNames=['v'; 'c'; '0'; '1'; '2'; '3'; '4'; '5'; '6'; '7'; '8'; '9'; 'A'; 'B'; 'D'; 'E'; 'F'; 'G'; 'H'; 'I'; 'J'; 'K'; 'L'; 'M'; 'N'; 'O'; 'P'; 'Q'; 'R'; 'S'; 'T'; 'U'; 'W'; 'X'; 'Y'; 'Z']  dspbaimage=dspba_prim.jpg  text=fprintf('Out%s', AdvDSPBChannelOutDisplay(latency));  style=Optimised  dataSignals=4  foldingEnabled=off  channels=1  sampleRate=200  packetBeginPresent=off  packetBeginEnabled=off  visibilities=dspba_ChannelOutVis(gcb)  latency=0  latencyCorrection=0  version=20141013
  Mult : DSPBAPrim/Mult  primtype=mult  nInputs=2  nOutputs=1  omode=Inherit via internal rule  otype=sfix(16)  scale=2^-15  rndmethod=Unbiased  factor=1  satmethod=Symmetric  shift_vec=[0 1 2 -1]  value=0  inPortNames=[' '; ' ';]  outPortNames=[' ']  dspbaimage=dspba_prim.jpg  text=fprintf('X');  style=Optimised  visibilities=8+2^18+2^19  floatPrecision=float32_m23  floatRounding=correct  advOptions=[]  version=20130115
  SynthesisInfo : DSPBAPrim/SynthesisInfo  primtype=synthinfo  nInputs=0  nOutputs=0  omode=Inherit via internal rule  otype=sfix(16)  scale=2^-15  rndmethod=Truncate  factor=1  satmethod=Symmetric  shift_vec=[0 1 2 -1]  value=99  inPortNames=[' '; ' ';]  outPortNames=[' ']  dspbaimage=dspba_prim_ctrl.jpg  text=fprintf('Style=%s', style);  style=Scheduled  visibilities=32768  constraintInUse=off  constraintRelation=>  constraintLimit=2  bitAccurate=off  version=20150220
  Valid_Out : Outport
  Channel_Out : Outport  Port=2
  A_k_j_Read_Address : Outport  Port=3
  A_k_Read_Address : Outport  Port=4
  Acc_Init_Out : Outport  Port=5
  Acc_Valid_Out : Outport  Port=6
  wires:
  ChannelIn/2 -> ChannelOut/2
  ChannelOut/4 -> A_k_Read_Address/1
  Valid_In/1 -> ChannelIn/1
  Row_Index/1 -> ChannelIn/3
  Channel_In/1 -> ChannelIn/2
  ChannelIn/1 -> ChannelOut/1
  Mult/1 -> Add/2
  ChannelIn/3 -> Add/1, ChannelOut/4
  ChannelOut/1 -> Valid_Out/1
  ChannelOut/3 -> A_k_j_Read_Address/1
  ChannelOut/2 -> Channel_Out/1
  ChannelIn/4 -> Mult/1
  Column/1 -> ChannelIn/4
  Row/1 -> ChannelIn/5
  ChannelIn/5 -> Mult/2
  Add/1 -> ChannelOut/3
  ChannelIn/6 -> ChannelOut/5
  ChannelIn/7 -> ChannelOut/6
  Acc_Init_In/1 -> ChannelIn/6
  Acc_Valid_In/1 -> ChannelIn/7
  ChannelOut/5 -> Acc_Init_Out/1
  ChannelOut/6 -> Acc_Valid_Out/1
